simulink library "AP_PitchController"  (R2024a)
settings: Solver=VariableStepAuto  StartTime=0.0  StopTime=10.0  RelTol=1e-3
undefined symbols (not defined in the file): PTCH2SRV_RLL, PTCH2SRV_TCONST, PTCH_Freq, PTCH_RATE_D, PTCH_RATE_I, PTCH_RATE_P, YAW_Freq
libraries: simulink_extras x4, ArdupilotFunctions x1
settings Model: Creator=igmso  LastModifiedBy=igmso

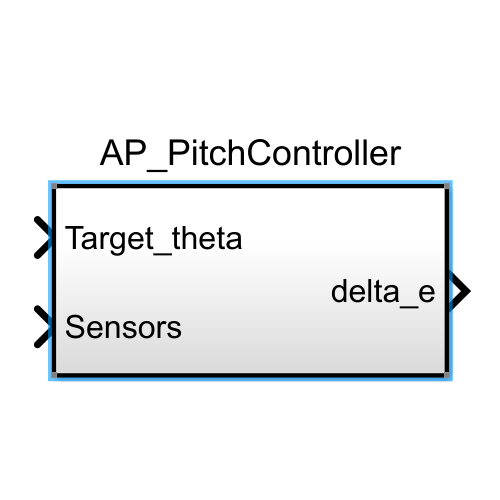
[thumbnail: Simulink's stored preview of the top-level diagram]
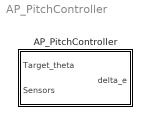
== system AP_PitchController ==
  AP_PitchController : Subsystem  TreatAsAtomicUnit=on  SystemSampleTime=1/PTCH_Freq

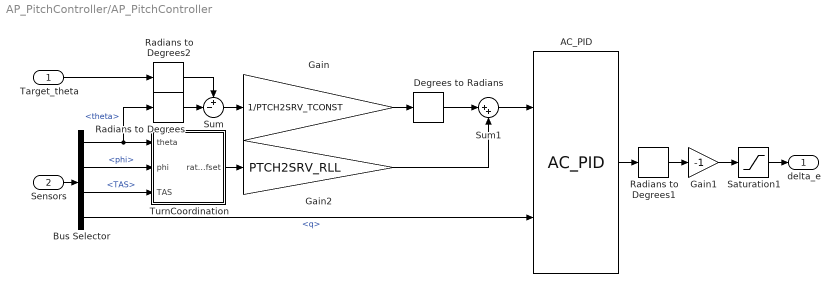
== system AP_PitchController/AP_PitchController ==
  Target_theta : Inport
  Sensors : Inport  Port=2
  AC_PID : ArdupilotFunctions/AC_PID  P=PTCH_RATE_P  I=PTCH_RATE_I  D=PTCH_RATE_D  FF=PTCH_RATE_FF  D_FF=PTCH_RATE_D_FF  FLTD=PTCH_RATE_FLTD  FLTE=PTCH_RATE_FLTE  FLTT=PTCH_RATE_FLTT  IMAX=PTCH_RATE_IMAX  ControlFreq=PTCH_Freq
  Bus Selector : BusSelector  OutputSignals=theta,phi,TAS,q
  Degrees to Radians : simulink_extras/Transformations/Degrees to Radians
  Gain : Gain  Gain=1/PTCH2SRV_TCONST
  Gain1 : Gain  Gain=-1
  Gain2 : Gain  Gain=PTCH2SRV_RLL
  Radians to Degrees : simulink_extras/Transformations/Radians to Degrees
  Radians to Degrees1 : simulink_extras/Transformations/Radians to Degrees
  Radians to Degrees2 : simulink_extras/Transformations/Radians to Degrees
  Saturation1 : Saturate  UpperLimit=45  LowerLimit=-45
  Sum : Sum  Inputs=+-|
  Sum1 : Sum  Inputs=|++
  TurnCoordination : Subsystem
  delta_e : Outport
  wires:
  Bus Selector/3 -> TurnCoordination/3(TAS)  "<TAS>"
  Gain2/1 -> Sum1/2
  TurnCoordination/1(rate_offset) -> Gain2/1
  Bus Selector/2 -> TurnCoordination/2(phi)  "<phi>"
  Sum1/1 -> AC_PID/1
  Radians to Degrees/1 -> Sum/2
  Degrees to Radians/1 -> Sum1/1
  Sensors/1 -> Bus Selector/1
  Bus Selector/1 -> TurnCoordination/1(theta), Radians to Degrees/1  "<theta>"
  Saturation1/1 -> delta_e/1
  Bus Selector/4 -> AC_PID/2  "<q>"
  AC_PID/1 -> Radians to Degrees1/1
  Sum/1 -> Gain/1
  Gain/1 -> Degrees to Radians/1
  Radians to Degrees2/1 -> Sum/1
  Gain1/1 -> Saturation1/1
  Radians to Degrees1/1 -> Gain1/1
  Target_theta/1 -> Radians to Degrees2/1

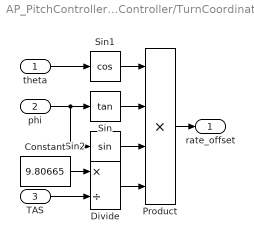
== system AP_PitchController/AP_PitchController/TurnCoordination ==
  theta : Inport
  phi : Inport  Port=2
  TAS : Inport  Port=3
  Constant : Constant  Value=9.80665  SampleTime=1/YAW_Freq
  Divide : Product  Inputs=*/
  Product : Product  Inputs=4
  Sin : Trigonometry  Operator=tan
  Sin1 : Trigonometry  Operator=cos
  Sin2 : Trigonometry
  rate_offset : Outport
  wires:
  Sin1/1 -> Product/1
  Sin2/1 -> Product/3
  theta/1 -> Sin1/1
  Constant/1 -> Divide/1
  phi/1 -> Sin/1, Sin2/1
  Sin/1 -> Product/2
  Product/1 -> rate_offset/1
  Divide/1 -> Product/4
  TAS/1 -> Divide/2
